simulink model "2_algorithm_DISS"  (R2020b)
settings: Solver=VariableStepAuto  StartTime=0.0  StopTime=10.0  RelTol=1e-3
undefined symbols (not defined in the file): deltaPsi, Psi, Vkx, Vkz
settings Model: Creator=Эрнест  LastModifiedBy=Эрнест

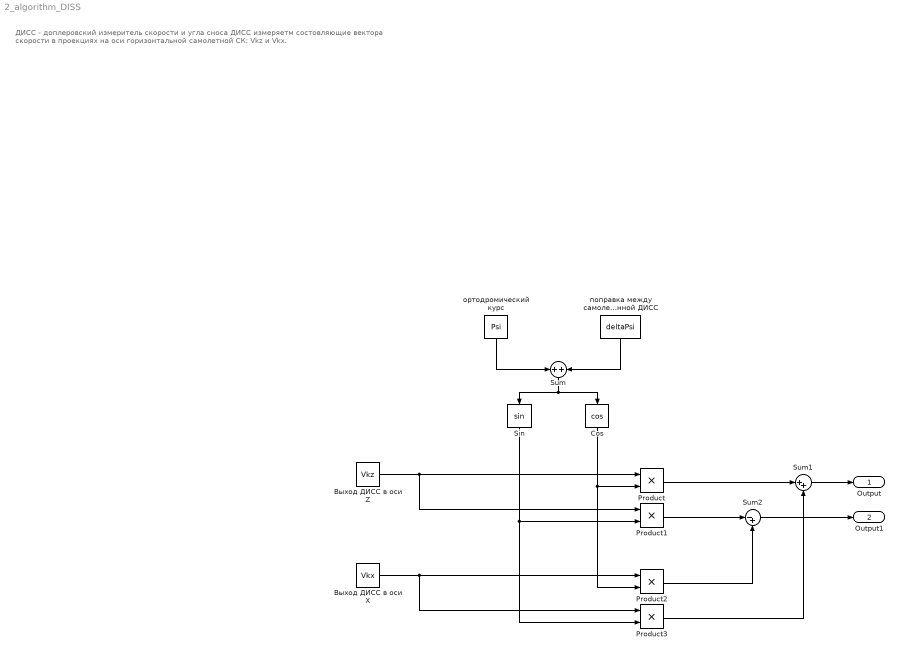
== system 2_algorithm_DISS ==
  note: ДИСС - доплеровский измеритель скорости и угла сноса
      |
      | ДИСС измеряетм состовляющие вектора скорости в проекциях на оси горизонтальной самолетной СК: Vkz и Vkx.
  Cos : Trigonometry  Operator=cos
  Product{,1..3} (4 alike) : Product
  Sin : Trigonometry
  Sum : Sum  Inputs=+|+
  Sum1 : Sum  Inputs=|++
  Sum2 : Sum  Inputs=|-+
  Выход ДИСС в оси X : Constant  Value=Vkx
  Выход ДИСС в оси Z : Constant  Value=Vkz
  ортодромический курс : Constant  Value=Psi
  "поправка между самолетной СК и СК, связанной с антенной ДИСС" : Constant  Value=deltaPsi
  Output : Outport
  Output1 : Outport  Port=2
  wires:
  "поправка между самолетной СК и СК, связанной с антенной ДИСС"/1 -> Sum/2
  ортодромический курс/1 -> Sum/1
  Sum/1 -> Cos/1, Sin/1
  Выход ДИСС в оси Z/1 -> Product1/1, Product/1
  Выход ДИСС в оси X/1 -> Product3/1, Product2/1
  Sin/1 -> Product3/2, Product1/2
  Cos/1 -> Product2/2, Product/2
  Product3/1 -> Sum1/2
  Product/1 -> Sum1/1
  Product1/1 -> Sum2/1
  Product2/1 -> Sum2/2
  Sum1/1 -> Output/1
  Sum2/1 -> Output1/1
